simulink library "TemperaturesJointChecker"  (R2016b)
settings: Solver=VariableStepAuto  StartTime=0.0  StopTime=10.0  RelTol=1e-3
undefined symbols (not defined in the file or in its folder): maxTemperatureJoint
settings Model: Creator=Nathan  LastModifiedBy=RKFE

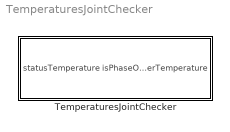
== system TemperaturesJointChecker ==
  TemperaturesJointChecker : Subsystem

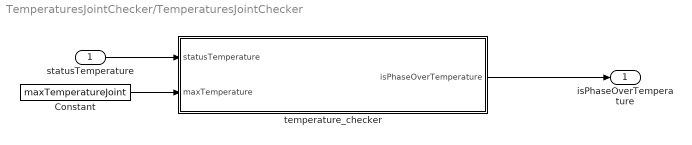
== system TemperaturesJointChecker/TemperaturesJointChecker ==
  statusTemperature : Inport  BusOutputAsStruct=on
  Constant : Constant  Value=maxTemperatureJoint  VectorParams1D=off  SampleTime=-1
  temperature_checker : MATLAB Function  TreatAsAtomicUnit=on
  isPhaseOverTemperature : Outport
  wires:
  statusTemperature/1 -> temperature_checker/1(statusTemperature)
  temperature_checker/1(isPhaseOverTemperature) -> isPhaseOverTemperature/1
  Constant/1 -> temperature_checker/2(maxTemperature)

== matlab function TemperaturesJointChecker/temperature_checker ==
  data: statusTemperature input; isPhaseOverTemperature output; maxTemperature input
function isPhaseOverTemperature = temperature_checker(statusTemperature,maxTemperature)


if(statusTemperature >= maxTemperature)
    isPhaseOverTemperature = 1;
    %Checks if the measured temperature does not exceed the maximum allowed
    %temperature
    
else
    isPhaseOverTemperature = 0;
end
